simulink model "sampleModel1817"  (R2023a)
settings: Solver=VariableStepAuto  StartTime=0.0  StopTime=10.0  RelTol=1e-3
libraries: hdlsllib x4, simulink x1
settings Model: Creator=user1  LastModifiedBy=user1

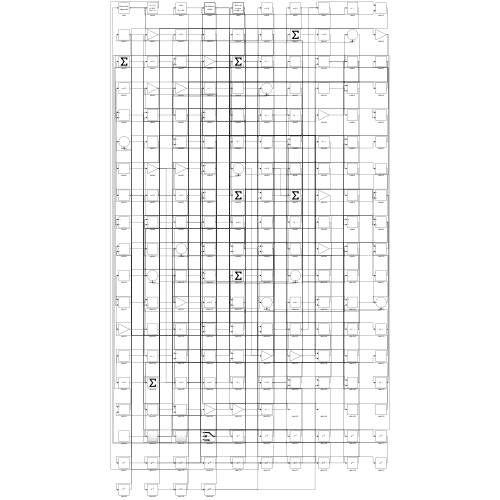
[thumbnail: Simulink's stored preview of the top-level diagram]
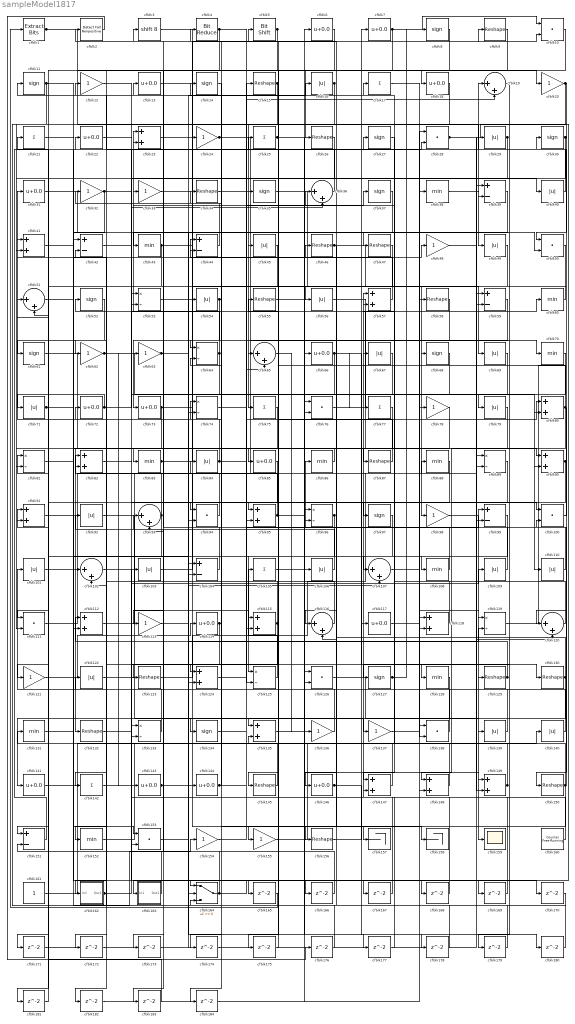
== system sampleModel1817 ==
  cfblk1 : simulink/Logic and Bit Operations/Extract Bits  bitsToExtract=Upper half  numBits=8  bitIdxRange=[0 7]  outScalingMode=Preserve fixed-point scaling
      settings: LibrarySourceBlock=|
      | hdlsllib/Logic and Bit
      | Operations/Extract Bits
  cfblk{10,28,50,76,94,100,111,126,138,153} (10 alike) : DotProduct  OutDataTypeStr=Inherit: Inherit via internal rule
  cfblk{16,29,40,45,49,54,56,67,69,71,79,84,92,101,103,106,109..110,122,139..140} (21 alike) : Abs  SaturateOnIntegerOverflow=off
  cfblk{19,36,51,65,93,102,107,116,120} (9 alike) : Sum  Inputs=|++
  cfblk{39,42,44,59,99,104,151} (7 alike) : Sum  Inputs=+-
  cfblk{17,21,25,75,77,105,142} (7 alike) : Sum  Inputs=+
  cfblk{38,43,60,70,83,86,88,108,128,131,152} (11 alike) : MinMax
  cfblk{8,11,14,27,30,35,37,52,61,68,97,127,134} (13 alike) : Signum
  cfblk{23,41,57,80,82,90..91,95,112,115,118,124,135,147..149} (16 alike) : Sum
  cfblk{12,20,24,32..33,48,62..63,78,98,113,121,136..137,154..155} (16 alike) : Gain
  cfblk{6..7,13,18,22,31,66,72..73,85,114,117,141,143..144,146} (16 alike) : Bias  Bias=0.0  SaturateOnIntegerOverflow=off
  cfblk{53,64,74,81,89,96,119,125,133} (9 alike) : Product  Inputs=*/  RndMeth=Zero  SaturateOnIntegerOverflow=on
  cfblk{9,15,26,34,46..47,55,58,87,123,129..130,132,145,150,156} (16 alike) : Reshape
  cfblk157 : Terminator
  cfblk158 : Terminator
  cfblk159 : Scope
  cfblk160 : hdlsllib/Sources/Counter Free-Running  NumBits=16  tsamp=-1
  cfblk161 : Constant  SampleTime=-1
  cfblk162 : Subsystem
      settings: LibrarySourceBlock=|
      | hdlsllib/Ports &
      | Subsystems/Subsystem
  cfblk163 : Subsystem
      settings: LibrarySourceBlock=|
      | hdlsllib/Ports &
      | Subsystems/Subsystem
  cfblk164 : Switch  SaturateOnIntegerOverflow=off  InputSameDT=off
  cfblk{165..184} (20 alike) : Delay  SampleTime=1
  cfblk2 : hdlsllib/Logic and Bit Operations/Detect Fall Nonpositive  vinit=0  OutDataTypeStr=boolean
  cfblk3 : ArithShift  BitShiftNumber=8
  cfblk4 : hdlsllib/Logic and Bit Operations/Bit Reduce  mode=AND
  cfblk5 : hdlsllib/Logic and Bit Operations/Bit Shift  mode=Shift Left Logical  N=0
  wires:
  cfblk65/1 -> cfblk136/1
  cfblk84/1 -> cfblk31/1, cfblk65/2
  cfblk91/1 -> cfblk70/1
  cfblk73/1 -> cfblk157/1, cfblk111/2
  cfblk60/1 -> cfblk56/1
  cfblk119/1 -> cfblk23/1
  cfblk104/1 -> cfblk52/1
  cfblk151/1 -> cfblk22/1
  cfblk160/1 -> cfblk57/1
  cfblk77/1 -> cfblk132/1
  cfblk23/1 -> cfblk158/1
  cfblk121/1 -> cfblk114/1
  cfblk122/1 -> cfblk137/1
  cfblk83/1 -> cfblk9/1, cfblk107/2
  cfblk64/1 -> cfblk23/2, cfblk173/1
  cfblk70/1 -> cfblk79/1
  cfblk102/1 -> cfblk135/1
  cfblk142/1 -> cfblk7/1
  cfblk37/1 -> cfblk43/1
  cfblk130/1 -> cfblk2/1, cfblk175/1
  cfblk46/1 -> cfblk98/1, cfblk156/1
  cfblk135/1 -> cfblk6/1
  cfblk28/1 -> cfblk163/1(In1), cfblk120/2
  cfblk75/1 -> cfblk164/1
  cfblk155/1 -> cfblk117/1
  cfblk32/1 -> cfblk53/1, cfblk112/2
  cfblk86/1 -> cfblk85/1
  cfblk18/1 -> cfblk75/1
  cfblk44/1 -> cfblk3/1
  cfblk127/1 -> cfblk17/1, cfblk8/1
  cfblk103/1 -> cfblk88/1
  cfblk120/1 -> cfblk33/1
  cfblk108/1 -> cfblk86/1
  cfblk74/1 -> cfblk15/1
  cfblk66/1 -> cfblk145/1, cfblk77/1, cfblk130/1
  cfblk96/1 -> cfblk125/1, cfblk123/1
  cfblk161/1 -> cfblk54/1
  cfblk145/1 -> cfblk122/1
  cfblk35/1 -> cfblk138/1
  cfblk1/1 -> cfblk49/1, cfblk95/2
  cfblk72/1 -> cfblk71/1, cfblk36/2, cfblk128/1
  cfblk9/1 -> cfblk26/1
  cfblk33/1 -> cfblk69/1
  cfblk53/1 -> cfblk16/1
  cfblk40/1 -> cfblk19/1
  cfblk89/1 -> cfblk148/1
  cfblk25/1 -> cfblk66/1, cfblk177/1
  cfblk56/1 -> cfblk90/1
  cfblk54/1 -> cfblk73/1, cfblk124/1, cfblk134/1
  cfblk10/1 -> cfblk18/1
  cfblk30/1 -> cfblk64/1, cfblk81/2
  cfblk34/1 -> cfblk68/1
  cfblk139/1 -> cfblk101/1
  cfblk141/1 -> cfblk29/1
  cfblk52/1 -> cfblk111/1
  cfblk150/1 -> cfblk5/1, cfblk100/2, cfblk184/1
  cfblk68/1 -> cfblk133/2
  cfblk61/1 -> cfblk87/1
  cfblk11/1 -> cfblk154/1, cfblk153/1, cfblk51/2
  cfblk45/1 -> cfblk53/2
  cfblk39/1 -> cfblk83/1
  cfblk98/1 -> cfblk159/1
  cfblk20/1 -> cfblk61/1, cfblk50/1
  cfblk126/1 -> cfblk139/1
  cfblk87/1 -> cfblk55/1
  cfblk5/1 -> cfblk182/1, cfblk183/1
  cfblk62/1 -> cfblk110/1, cfblk143/1, cfblk60/1
  cfblk24/1 -> cfblk118/2, cfblk50/2
  cfblk36/1 -> cfblk12/1
  cfblk85/1 -> cfblk151/1
  cfblk115/1 -> cfblk41/1, cfblk172/1
  cfblk105/1 -> cfblk106/1
  cfblk16/1 -> cfblk95/1, cfblk125/2
  cfblk134/1 -> cfblk80/1
  cfblk100/1 -> cfblk30/1
  cfblk6/1 -> cfblk121/1
  cfblk80/1 -> cfblk44/1, cfblk120/1, cfblk108/1
  cfblk152/1 -> cfblk35/1
  cfblk26/1 -> cfblk63/1
  cfblk31/1 -> cfblk144/1
  cfblk48/1 -> cfblk39/1
  cfblk79/1 -> cfblk89/2
  cfblk123/1 -> cfblk38/1
  cfblk110/1 -> cfblk32/1
  cfblk146/1 -> cfblk10/2, cfblk178/1
  cfblk55/1 -> cfblk100/1
  cfblk117/1 -> cfblk119/1
  cfblk124/1 -> cfblk19/2
  cfblk125/1 -> cfblk105/1
  cfblk58/1 -> cfblk164/2
  cfblk118/1 -> cfblk11/1
  cfblk133/1 -> cfblk72/1
  cfblk42/1 -> cfblk27/1
  cfblk113/1 -> cfblk46/1
  cfblk13/1 -> cfblk20/1
  cfblk149/1 -> cfblk36/1, cfblk131/1
  cfblk94/1 -> cfblk42/2
  cfblk147/1 -> cfblk96/2
  cfblk59/1 -> cfblk116/1
  cfblk63/1 -> cfblk13/1, cfblk25/1
  cfblk3/1 -> cfblk76/1
  cfblk163/1(Out1) -> cfblk82/1
  cfblk57/1 -> cfblk34/1
  cfblk69/1 -> cfblk155/1
  cfblk111/1 -> cfblk59/2
  cfblk101/1 -> cfblk24/1
  cfblk143/1 -> cfblk48/1, cfblk119/2, cfblk180/1
  cfblk164/1 -> cfblk93/1, cfblk168/1
  cfblk140/1 -> cfblk91/1
  cfblk92/1 -> cfblk115/1
  cfblk162/1(Out1) -> cfblk109/1, cfblk166/1
  cfblk95/1 -> cfblk14/1, cfblk64/2, cfblk149/1
  cfblk8/1 -> cfblk45/1
  cfblk99/1 -> cfblk107/1
  cfblk51/1 -> cfblk102/1
  cfblk93/1 -> cfblk82/2, cfblk153/2
  cfblk129/1 -> cfblk127/1, cfblk112/1
  cfblk107/1 -> cfblk78/1
  cfblk114/1 -> cfblk84/1, cfblk124/2
  cfblk90/1 -> cfblk129/1, cfblk150/1, cfblk149/2
  cfblk4/1 -> cfblk162/1(In1), cfblk126/2, cfblk99/2
  cfblk106/1 -> cfblk92/1
  cfblk22/1 -> cfblk97/1
  cfblk112/1 -> cfblk76/2
  cfblk21/1 -> cfblk47/1
  cfblk132/1 -> cfblk103/1
  cfblk7/1 -> cfblk10/1, cfblk65/1
  cfblk17/1 -> cfblk80/2
  cfblk128/1 -> cfblk141/1
  cfblk43/1 -> cfblk138/2, cfblk142/1
  cfblk14/1 -> cfblk94/1
  cfblk116/1 -> cfblk4/1
  cfblk27/1 -> cfblk147/1
  cfblk49/1 -> cfblk113/1
  cfblk88/1 -> cfblk152/1
  cfblk154/1 -> cfblk37/1
  cfblk148/1 -> cfblk57/2
  cfblk137/1 -> cfblk58/1
  cfblk29/1 -> cfblk115/2, cfblk93/2
  cfblk38/1 -> cfblk39/2
  cfblk15/1 -> cfblk41/2, cfblk62/1
  cfblk78/1 -> cfblk146/1
  cfblk12/1 -> cfblk40/1
  cfblk76/1 -> cfblk28/1
  cfblk156/1 -> cfblk140/1
  cfblk71/1 -> cfblk104/2, cfblk90/2
  cfblk136/1 -> cfblk21/1
  cfblk131/1 -> cfblk28/2
  cfblk138/1 -> cfblk81/1
  cfblk109/1 -> cfblk67/1
  cfblk144/1 -> cfblk74/1, cfblk99/1
  cfblk41/1 -> cfblk44/2
  cfblk67/1 -> cfblk165/1
  cfblk165/1 -> cfblk1/1
  cfblk166/1 -> cfblk91/2
  cfblk81/1 -> cfblk167/1
  cfblk167/1 -> cfblk133/1
  cfblk168/1 -> cfblk104/1
  cfblk82/1 -> cfblk169/1
  cfblk169/1 -> cfblk89/1
  cfblk153/1 -> cfblk170/1
  cfblk170/1 -> cfblk164/3
  cfblk47/1 -> cfblk171/1
  cfblk171/1 -> cfblk148/2
  cfblk172/1 -> cfblk74/2
  cfblk173/1 -> cfblk94/2
  cfblk50/1 -> cfblk174/1
  cfblk174/1 -> cfblk59/1
  cfblk175/1 -> cfblk135/2
  cfblk2/1 -> cfblk176/1
  cfblk176/1 -> cfblk42/1
  cfblk177/1 -> cfblk147/2
  cfblk178/1 -> cfblk96/1
  cfblk19/1 -> cfblk179/1
  cfblk179/1 -> cfblk116/2
  cfblk180/1 -> cfblk102/2
  cfblk97/1 -> cfblk181/1
  cfblk181/1 -> cfblk151/2
  cfblk182/1 -> cfblk118/1
  cfblk183/1 -> cfblk51/1
  cfblk184/1 -> cfblk126/1

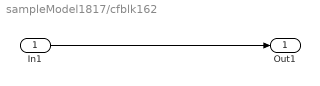
== system sampleModel1817/cfblk162 ==
  In1 : Inport
  Out1 : Outport
  wires:
  In1/1 -> Out1/1

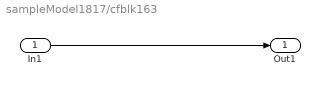
== system sampleModel1817/cfblk163 ==
  In1 : Inport
  Out1 : Outport
  wires:
  In1/1 -> Out1/1
